simulink model "modelo_completo_codesys_final"  (R2020a)
settings: Solver=FixedStepAuto  StartTime=0.0  StopTime=inf  FixedStep=0.5e-3  MaxStep=1e-3  RelTol=1e-3
undefined symbols (not defined in the file): bac, baiz, bcx, bcy, Beqtran, Bheqd, bw, DiscIntNeverNeededParam, g, Kcy, ksac, ksaiz, ksiac, ksiaiz, Kw, lh0, Meq, Mheq, Rd, Rr, rt, rtd, xl0, xt0, yl0, yt0
libraries: simulink x13, powerlib_meascontrol x4, vrlib x2, dspswit3 x1
settings Model: SimulationMode=accelerator  Creator=tomas  LastModifiedBy=quiro
settings DataIOCC: ReturnWorkspaceOutputs=off
settings OptimizationCC: EfficientMapNaN2IntZero=off
settings DebuggingCC: ArithmeticOperatorsInVariantConditions=warning
settings HardwareCC: ProdBitPerPointer=32  ProdBitPerSizeT=32  ProdBitPerPtrDiffT=32  ProdWordSize=32  ProdHWDeviceType=Intel->x86-32 (Windows32)  TargetBitPerPointer=64  TargetBitPerSizeT=64  TargetBitPerPtrDiffT=64  TargetLongLongMode=on  TargetIntDivRoundTo=Zero  TargetEndianess=LittleEndian  TargetWordSize=64  TargetHWDeviceType=MATLAB Host  ProdEqTarget=off
settings SFSimCC: SimUseLocalCustomCode=off  CustomCodeUndefinedFunction=UseInterfaceOnly
settings RTWCC: RTWUseLocalCustomCode=off
settings CodeAppCC: MaxIdLength=128  StateflowObjectComments=on
settings GRTTargetCC: TargetLangStandard=C89/C90 (ANSI)  CombineOutputUpdateFcns=off  GRTInterface=on
settings SimscapeCC: SimscapeNormalizeSystem=off

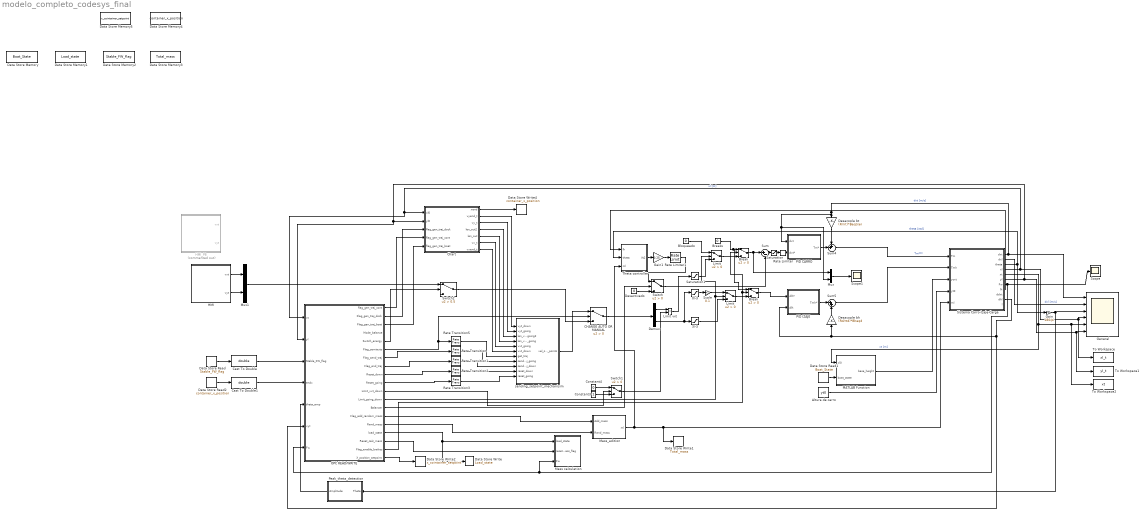
== system modelo_completo_codesys_final ==
  0/-3 : Saturate  UpperLimit=0.0  LowerLimit=-3.0
  3/-3 : Saturate  UpperLimit=3.0  LowerLimit=-3.0
  Altura de carro : Constant  Value=yt0
  Bloqueado : Constant  Value=0
  Break : Switch  Criteria=u2 > Threshold
  "Break " : Switch  Criteria=u2 > Threshold
  Breaks : Constant  Value=0
  CHANGE AUTO OR MANUAL : Switch  Criteria=u2 > Threshold
  Cast To Double : DataTypeConversion  OutDataTypeStr=double
  Cast To Double1 : DataTypeConversion  OutDataTypeStr=double
  Chart : Stateflow chart  TreatAsAtomicUnit=on
      settings: PortSchema="{\"entries\":[{\"content\":{\"sides\":[{\"content\":{\"connectorIds\":[\"In1\",\"In2\",\"In4\",\"In5\",\"In3\"]},\"type\":\"ConnectorPlacement.EquallySpacedRectSide\",\"uuid\":\"6b1ea9ed-88c8-4f45-af53-cf9c910626a6\"},{\"content\":{\"connectorIds\":[\"Out1\",\"Out2\",\"Out3\",\"Out4\",\"Out5\",\"Out6\",\"Out7\"],\"side\":\"RIGHT\"},\"type\":\"ConnectorPlacement.EquallySpacedRectSide\",\"uuid\":\"2b247f2b-a163-4c54-9e4e-ffcd144f96a2\"},{\"content\":{\"connectorIds\":[],\"side\":\"TOP\"},\"type\":\"ConnectorPlacement.EquallySpacedRectSide\",\"uuid\":\"aad476ba-6ce1-4a52-a412-e890bbacaba3\"}]},\"type\":\"ConnectorPlacement.EquallySpacedConnector\",\"uuid\":\"baf22a08-585d-4fcd-a6c0-f3cd3f47f06b\"}],\"packageUris\":[\"http://schema.mathworks.com/mf0/Connector/19700101\"],\"version\":\"1.0\"}"
  Constant3 : Constant
  Constant4 : Constant  Value=0
  Data Store Memory : DataStoreMemory  DataStoreName=Boat_State  ReadBeforeWriteMsg=warning  WriteAfterWriteMsg=warning  WriteAfterReadMsg=warning  InitialValue=[6;5;7;4;5; 4]  ShowAdditionalParam=off  OutDataTypeStr=double
  Data Store Memory1 : DataStoreMemory  DataStoreName=Load_state  ReadBeforeWriteMsg=warning  WriteAfterWriteMsg=warning  WriteAfterReadMsg=warning  ShowAdditionalParam=off  OutDataTypeStr=double
  Data Store Memory2 : DataStoreMemory  DataStoreName=Stable_FW_flag  ReadBeforeWriteMsg=warning  WriteAfterWriteMsg=warning  WriteAfterReadMsg=warning  ShowAdditionalParam=off  OutDataTypeStr=boolean
  Data Store Memory3 : DataStoreMemory  DataStoreName=Total_mass  ReadBeforeWriteMsg=warning  WriteAfterWriteMsg=warning  WriteAfterReadMsg=warning  InitialValue=15000.0  ShowAdditionalParam=off  OutDataTypeStr=double
  Data Store Memory4 : DataStoreMemory  DataStoreName=container_x_position  ReadBeforeWriteMsg=warning  WriteAfterWriteMsg=warning  WriteAfterReadMsg=warning  InitialValue=0.0  ShowAdditionalParam=off  OutDataTypeStr=double
  Data Store Memory5 : DataStoreMemory  DataStoreName=x_cointainer_setpoint  ReadBeforeWriteMsg=warning  WriteAfterWriteMsg=warning  WriteAfterReadMsg=warning  InitialValue=4  ShowAdditionalParam=off  OutDataTypeStr=double
  Data Store Read : DataStoreRead  DataStoreName=Stable_FW_flag
  Data Store Read1 : DataStoreRead  DataStoreName=Boat_State
  Data Store Read2 : DataStoreRead  DataStoreName=container_x_position  SampleTime=0.1
  Data Store Write : DataStoreWrite  DataStoreName=Load_state
  Data Store Write1 : DataStoreWrite  DataStoreName=Total_mass
  Data Store Write2 : DataStoreWrite  DataStoreName=x_cointainer_setpoint
  Data Store Write4 : DataStoreWrite  DataStoreName=container_x_position
  Demux : Demux  Outputs=2
  Desacople bh : Gain  Gain=(Rd/rtd)*Bheqd
  Desacople bt : Gain  Gain=(Rr/rt)*Beqtran
  Desactivado : Constant  Value=0
  Gain : Gain  Gain=180/pi
  Gain1 : Gain  Gain=0.25
  General : Scope  NumInputPorts=6
  HMI : Subsystem
  HMI_P8 : Subsystem  Commented=on
  Limit : Switch  Criteria=u2 > Threshold
  "Limit " : Switch  Criteria=u2 > Threshold
  Limit vxt : Product
  MATLAB Function : MATLAB Function  TreatAsAtomicUnit=on
  Mass calculation : Subsystem
  Mass_adition : Subsystem
  Mux : Mux  Inputs=2
  Mux1 : Mux  Inputs=2
  OPC READ/WRITE : Subsystem  TreatAsAtomicUnit=on  SystemSampleTime=0.1
  "PID CARRO " : Subsystem
  PID IZAJE : Subsystem
  Peak_theta_detection : Subsystem
  Rate Limiter : RateLimiter  SampleTimeMode=inherited
  Rate Limiter1 : RateLimiter  SampleTimeMode=inherited
  Rate Transition{,1..3,5} (5 alike) : RateTransition
  Saturation : Saturate  UpperLimit=4  LowerLimit=-4
  Saturation1 : Saturate  UpperLimit=4.0  LowerLimit=-4.0
  Scale : Gain  Gain=0.1
  Scope : Scope
  Scope1 : Scope
  "Sistema Carro-Izaje-Carga " : Subsystem
  Sum : Sum  Inputs=|+-
  Sum4 : Sum  Inputs=++|
  Sum5 : Sum  Inputs=|++
  Switch : Switch  Criteria=u2 > Threshold
  Switch1 : Switch  Criteria=u2 > Threshold
  Switch2 : Switch  Criteria=u2 > Threshold  Threshold=0.5
  Theta controller : Subsystem
  To Workspace : ToWorkspace  VariableName=xl_t  SampleTime=-1
  To Workspace1 : ToWorkspace  VariableName=yl_t  SampleTime=-1
  To Workspace2 : ToWorkspace  VariableName=xt  SampleTime=-1
  sending_setpoint_mechanisim : Subsystem
  wires:
  Sum4/1 -> "Sistema Carro-Izaje-Carga "/1(Tm)  "Tm***"
  Desacople bt/1 -> Sum4/1
  Desacople bh/1 -> Sum5/2
  PID IZAJE/1("Tmh* ") -> Sum5/1
  Switch/1 -> Sum/2
  Sum5/1 -> "Sistema Carro-Izaje-Carga "/2(Tmh)
  MATLAB Function/1(base_height) -> "Sistema Carro-Izaje-Carga "/3(ycxt)
  Altura de carro/1 -> "Sistema Carro-Izaje-Carga "/4(yt0)
  "Sistema Carro-Izaje-Carga "/1(dxt) -> General/1, "PID CARRO "/1(dxt), Mux/2, Desacople bt/1  "dxt [m/s]"
  "Sistema Carro-Izaje-Carga "/10(dhl) -> OPC READ/WRITE/6(vyt), PID IZAJE/2(dlh), Desacople bh/1
  Desactivado/1 -> Switch/3
  "Sistema Carro-Izaje-Carga "/8(lh) -> Theta controller/1(lh)
  "Sistema Carro-Izaje-Carga "/2(dxl) -> General/2  "dxl [m/s]"
  "Sistema Carro-Izaje-Carga "/3(theta) -> Theta controller/2(theta), Gain/1  "theta [rad]"
  "Sistema Carro-Izaje-Carga "/4(xl) -> OPC READ/WRITE/1(xt), Chart/1(xl0), General/4, To Workspace/1  "xl [m]"
  "Sistema Carro-Izaje-Carga "/5(xt) -> MATLAB Function/1(xl0), To Workspace2/1, General/5  "xt [m]"
  "PID CARRO "/1(Tm*) -> Sum4/2
  Gain/1 -> General/3, Peak_theta_detection/1(Theta)
  OPC READ/WRITE/13(Balancer) -> Switch/2
  HMI/1(vxt) -> Mux1/1
  HMI/2(vyt) -> Mux1/2
  OPC READ/WRITE/6(Flag_semiauto) -> CHANGE AUTO OR MANUAL/2, Rate Transition5/1
  CHANGE AUTO OR MANUAL/1 -> Demux/1
  Demux/2 -> 3/-3/1, 0/-3/1
  Peak_theta_detection/1(Amplitude) -> OPC READ/WRITE/5(theta_amp)
  OPC READ/WRITE/7(Flag_send_traj) -> Rate Transition/1
  OPC READ/WRITE/8(Flag_end_traj) -> Rate Transition1/1
  sending_setpoint_mechanisim/1(vel_sets_points) -> CHANGE AUTO OR MANUAL/1
  OPC READ/WRITE/10(Reset_going) -> Rate Transition3/1
  OPC READ/WRITE/9(Reset_down) -> Rate Transition2/1
  Saturation1/1 -> Limit/3
  "Limit "/1 -> "Break "/3
  0/-3/1 -> Scale/1
  Limit/1 -> Break/3
  Bloqueado/1 -> Limit/1
  Scale/1 -> "Limit "/1
  3/-3/1 -> "Limit "/3
  "Sistema Carro-Izaje-Carga "/7(Fw) -> Mass calculation/3(Fw), OPC READ/WRITE/7(Fw), Scope/1
  OPC READ/WRITE/11(Limit_vxt_down) -> Switch1/2
  Constant3/1 -> Switch1/3
  Constant4/1 -> Switch1/1
  Demux/1 -> Limit vxt/1
  Switch1/1 -> Limit vxt/2
  Limit vxt/1 -> Saturation1/1
  Data Store Read1/1 -> MATLAB Function/2(boat_state)
  Mass_adition/1(ml) -> Theta controller/3(ml), "Sistema Carro-Izaje-Carga "/5(ml), Data Store Write1/1
  OPC READ/WRITE/14(Flag_add_random_mass) -> Mass_adition/1(Add_mass)
  OPC READ/WRITE/15(Rand_mass) -> Mass_adition/2(Rand_mass)
  OPC READ/WRITE/17(Reset_calc_mass) -> Mass calculation/2(reset_mass_flag)
  Break/1 -> Mux/1, Sum/1
  "Break "/1 -> PID IZAJE/1(dlh*)
  Breaks/1 -> "Break "/1, Break/1
  OPC READ/WRITE/12(Limit_going_down) -> Limit/2, "Limit "/2
  Chart/6(vx_t) -> sending_setpoint_mechanisim/5(vxt_going)
  Chart/7(vxend_t) -> sending_setpoint_mechanisim/6(vxt_down)
  Chart/3(vy_t) -> sending_setpoint_mechanisim/2(vyt_going)
  Chart/2(vyend_t) -> sending_setpoint_mechanisim/1(vyt_down)
  Chart/4(len_out2) -> sending_setpoint_mechanisim/3(len_vec_going2)
  Chart/5(len_out) -> sending_setpoint_mechanisim/4(len_vec_going)
  OPC READ/WRITE/3(Flag_gen_traj_boat) -> Chart/3(flag_gen_traj_boat)
  OPC READ/WRITE/2(Flag_gen_traj_dock) -> Chart/4(flag_gen_traj_dock)
  "Sistema Carro-Izaje-Carga "/6(yl) -> General/6, To Workspace1/1, OPC READ/WRITE/2(yl), Chart/2(yl0)
  Data Store Read/1 -> Cast To Double/1
  Cast To Double/1 -> OPC READ/WRITE/3(Stable_FW_flag)
  Rate Transition/1 -> sending_setpoint_mechanisim/8(send_traj_going)
  Rate Transition1/1 -> sending_setpoint_mechanisim/9(send_traj_down)
  Rate Transition2/1 -> sending_setpoint_mechanisim/10(reset_down)
  Rate Transition3/1 -> sending_setpoint_mechanisim/11(reset_going)
  Rate Transition5/1 -> sending_setpoint_mechanisim/7(get_traj)
  Chart/1(xend) -> Data Store Write4/1
  Data Store Read2/1 -> Cast To Double1/1
  Cast To Double1/1 -> OPC READ/WRITE/4(endx)
  OPC READ/WRITE/18(Flag_enable_brakes) -> "Break "/2, Break/2
  OPC READ/WRITE/16(load_state) -> Data Store Write/1, Mass calculation/1(load_state)
  Switch2/1 -> CHANGE AUTO OR MANUAL/3
  Mux1/1 -> Switch2/1
  OPC READ/WRITE/5(Switch_energy) -> Switch2/2
  OPC READ/WRITE/19(X_position_setpoint) -> Data Store Write2/1
  OPC READ/WRITE/1(flag_gen_traj_cont) -> Chart/5(flag_gen_traj_cont)
  Gain1/1 -> Rate Limiter1/1
  Theta controller/1(Vt2) -> Gain1/1
  Rate Limiter1/1 -> Switch/1
  Sum/1 -> Saturation/1
  Saturation/1 -> Rate Limiter/1
  Rate Limiter/1 -> "PID CARRO "/2(dxt*)
  Mux/1 -> Scope1/1

== system modelo_completo_codesys_final/HMI ==
  Demux : Demux  Outputs=3
  First-Order Filter : powerlib_meascontrol/Filters/First-Order Filter  FilterType=Lowpass  Tc=10e-3  Ts=0  Initialize=off  Vac_Init=[0, 0, 60]  Vdc_Init=0  PlotResponse=off  FreqRange="[0,  200,  1]"
  First-Order Filter1 : powerlib_meascontrol/Filters/First-Order Filter  FilterType=Lowpass  Tc=10e-3  Ts=0  Initialize=off  Vac_Init=[0, 0, 60]  Vdc_Init=0  PlotResponse=off  FreqRange="[0,  200,  1]"
  Joystick Input : vrlib/Joystick Input  joyid=1  adjustports=on  forcefeed=off
  vxt : Outport
  vyt : Outport  Port=2
  wires:
  First-Order Filter1/1 -> vyt/1
  First-Order Filter/1 -> vxt/1
  Joystick Input/1 -> Demux/1
  Demux/1 -> First-Order Filter/1
  Demux/2 -> First-Order Filter1/1

== system modelo_completo_codesys_final/HMI_P8 ==
  Demux : Demux  Outputs=3
  Demux1 : Demux  Commented=on  Outputs=12
  First-Order Filter : powerlib_meascontrol/Filters/First-Order Filter  FilterType=Lowpass  Tc=10e-3  Ts=0  Initialize=off  Vac_Init=[0, 0, 60]  Vdc_Init=0  PlotResponse=off  FreqRange="[0,  200,  1]"
  First-Order Filter1 : powerlib_meascontrol/Filters/First-Order Filter  FilterType=Lowpass  Tc=10e-3  Ts=0  Initialize=off  Vac_Init=[0, 0, 60]  Vdc_Init=0  PlotResponse=off  FreqRange="[0,  200,  1]"
  Joystick Input : vrlib/Joystick Input  joyid=1  adjustports=on  forcefeed=off
  Scope : Scope  Commented=on  NumInputPorts=12
  Scope1 : Scope  NumInputPorts=2
  vxt : Outport
  vyt : Outport  Port=2
  wires:
  Joystick Input/1 -> Demux/1
  Demux1/12 -> Scope/12
  Demux1/11 -> Scope/11
  Demux1/10 -> Scope/10
  Demux1/9 -> Scope/9
  Demux1/8 -> Scope/8
  Demux1/7 -> Scope/7
  Demux1/6 -> Scope/6
  Demux1/5 -> Scope/5
  Demux1/4 -> Scope/4
  Demux1/3 -> Scope/3
  Demux1/2 -> Scope/2
  Demux1/1 -> Scope/1
  Demux/3 -> First-Order Filter1/1
  Demux/2 -> First-Order Filter/1
  Joystick Input/2 -> Demux1/1
  First-Order Filter/1 -> vxt/1, Scope1/1
  First-Order Filter1/1 -> vyt/1, Scope1/2

== system modelo_completo_codesys_final/Mass calculation ==
  load_state : Inport
  reset_mass_flag : Inport  Port=2
  Fw : Inport  Port=3
  Subsystem : Subsystem
  Subsystem1 : Subsystem
  wires:
  Fw/1 -> Subsystem1/1(Fw), Subsystem/1(Fw)
  load_state/1 -> Subsystem/Enable
  reset_mass_flag/1 -> Subsystem1/Enable, Subsystem/2(In1)

== system modelo_completo_codesys_final/Mass_adition ==
  Add_mass : Inport
  Rand_mass : Inport  Port=2
  Constant : Constant  Value=0
  Constant2 : Constant  Value=15000
  Sum1 : Sum
  add_random_mass : Switch  Criteria=u2 > Threshold
  ml : Outport
  wires:
  Add_mass/1 -> add_random_mass/2
  Constant/1 -> add_random_mass/3
  add_random_mass/1 -> Sum1/2
  Constant2/1 -> Sum1/1
  Sum1/1 -> ml/1
  Rand_mass/1 -> add_random_mass/1

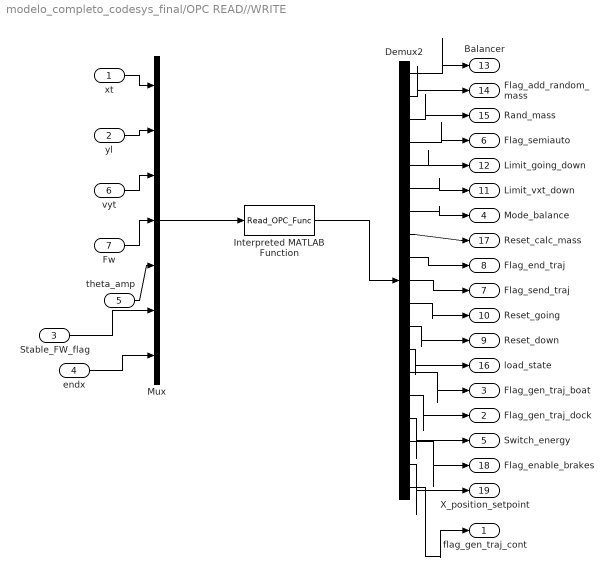
== system modelo_completo_codesys_final/OPC READ//WRITE ==
  xt : Inport
  yl : Inport  Port=2
  Stable_FW_flag : Inport  Port=3
  endx : Inport  Port=4
  theta_amp : Inport  Port=5
  vyt : Inport  Port=6
  Fw : Inport  Port=7
  Demux2 : Demux  Outputs=19
  Interpreted MATLAB Function : MATLABFcn  MATLABFcn=Read_OPC_Func
  Mux : Mux  Inputs=7
  flag_gen_traj_cont : Outport
  Flag_gen_traj_dock : Outport  Port=2
  Flag_gen_traj_boat : Outport  Port=3
  Mode_balance : Outport  Port=4
  Switch_energy : Outport  Port=5
  Flag_semiauto : Outport  Port=6
  Flag_send_traj : Outport  Port=7
  Flag_end_traj : Outport  Port=8
  Reset_down : Outport  Port=9
  Reset_going : Outport  Port=10
  Limit_vxt_down : Outport  Port=11
  Limit_going_down : Outport  Port=12
  Balancer : Outport  Port=13
  Flag_add_random_mass : Outport  Port=14
  Rand_mass : Outport  Port=15
  load_state : Outport  Port=16
  Reset_calc_mass : Outport  Port=17
  Flag_enable_brakes : Outport  Port=18
  X_position_setpoint : Outport  Port=19
  wires:
  Interpreted MATLAB Function/1 -> Demux2/1
  Stable_FW_flag/1 -> Mux/6
  Demux2/13 -> load_state/1
  Demux2/2 -> Flag_add_random_mass/1
  Demux2/12 -> Reset_down/1
  Demux2/11 -> Reset_going/1
  Demux2/9 -> Flag_end_traj/1
  Demux2/7 -> Mode_balance/1
  Demux2/3 -> Rand_mass/1
  Demux2/5 -> Limit_going_down/1
  Demux2/6 -> Limit_vxt_down/1
  Demux2/1 -> Balancer/1
  yl/1 -> Mux/2
  Mux/1 -> Interpreted MATLAB Function/1
  xt/1 -> Mux/1
  Demux2/8 -> Reset_calc_mass/1
  vyt/1 -> Mux/3
  Demux2/10 -> Flag_send_traj/1
  theta_amp/1 -> Mux/5
  Fw/1 -> Mux/4
  Demux2/4 -> Flag_semiauto/1
  Demux2/14 -> Flag_gen_traj_boat/1
  Demux2/15 -> Flag_gen_traj_dock/1
  endx/1 -> Mux/7
  Demux2/16 -> Switch_energy/1
  Demux2/17 -> Flag_enable_brakes/1
  Demux2/18 -> X_position_setpoint/1
  Demux2/19 -> flag_gen_traj_cont/1

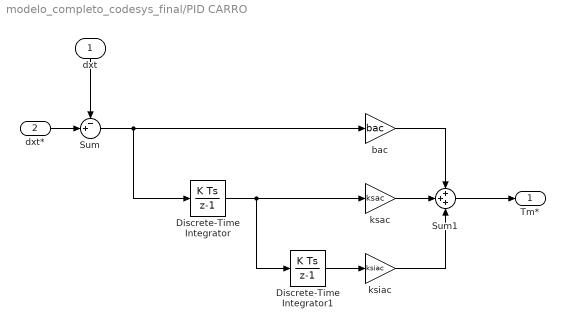
== system modelo_completo_codesys_final/PID CARRO  ==
  dxt : Inport
  dxt* : Inport  Port=2
  Discrete-Time Integrator : DiscreteIntegrator  SampleTime=-1  ICPrevOutput=DiscIntNeverNeededParam  ICPrevScaledInput=DiscIntNeverNeededParam
  Discrete-Time Integrator1 : DiscreteIntegrator  SampleTime=-1  ICPrevOutput=DiscIntNeverNeededParam  ICPrevScaledInput=DiscIntNeverNeededParam
  Sum : Sum  Inputs=-+|
  Sum1 : Sum  Inputs=+++
  bac : Gain  Gain=bac
  ksac : Gain  Gain=ksac
  ksiac : Gain  Gain=ksiac
  Tm* : Outport
  wires:
  dxt*/1 -> Sum/2
  dxt/1 -> Sum/1
  Sum1/1 -> Tm*/1
  bac/1 -> Sum1/1
  ksac/1 -> Sum1/2
  Discrete-Time Integrator1/1 -> ksiac/1
  ksiac/1 -> Sum1/3
  Sum/1 -> Discrete-Time Integrator/1, bac/1
  Discrete-Time Integrator/1 -> Discrete-Time Integrator1/1, ksac/1

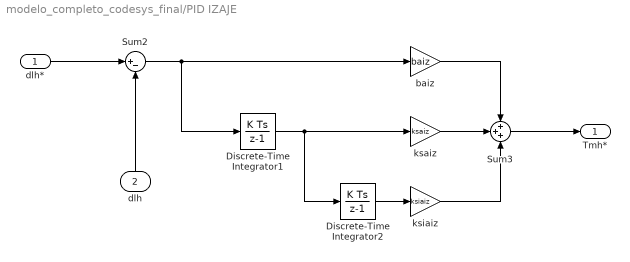
== system modelo_completo_codesys_final/PID IZAJE ==
  dlh* : Inport
  dlh : Inport  Port=2
  Discrete-Time Integrator1 : DiscreteIntegrator  SampleTime=-1  ICPrevOutput=DiscIntNeverNeededParam  ICPrevScaledInput=DiscIntNeverNeededParam
  Discrete-Time Integrator2 : DiscreteIntegrator  SampleTime=-1  ICPrevOutput=DiscIntNeverNeededParam  ICPrevScaledInput=DiscIntNeverNeededParam
  Sum2 : Sum  Inputs=|+-
  Sum3 : Sum  Inputs=+++
  baiz : Gain  Gain=baiz
  ksaiz : Gain  Gain=ksaiz
  ksiaiz : Gain  Gain=ksiaiz
  "Tmh* " : Outport
  wires:
  dlh/1 -> Sum2/2
  Sum3/1 -> "Tmh* "/1
  ksaiz/1 -> Sum3/2
  Discrete-Time Integrator2/1 -> ksiaiz/1
  baiz/1 -> Sum3/1
  ksiaiz/1 -> Sum3/3
  dlh*/1 -> Sum2/1
  Sum2/1 -> Discrete-Time Integrator1/1, baiz/1
  Discrete-Time Integrator1/1 -> Discrete-Time Integrator2/1, ksaiz/1

== system modelo_completo_codesys_final/Peak_theta_detection ==
  Theta : Inport
  Detect Decrease : simulink/Logic and Bit Operations/Detect Decrease  vinit=0.0  OutDataTypeStr=boolean
  Detect Rise Positive : simulink/Logic and Bit Operations/Detect Rise Positive  vinit=0  OutDataTypeStr=boolean
  MinMax Running Resettable : simulink/Math Operations/MinMax Running Resettable  Function=max  vinit=0.0
  Subsystem : Subsystem
  Amplitude : Outport
  wires:
  Theta/1 -> Detect Decrease/1, Detect Rise Positive/1, MinMax Running Resettable/1
  Subsystem/1(Out1) -> Amplitude/1
  MinMax Running Resettable/1 -> Subsystem/1(In1)
  Detect Rise Positive/1 -> MinMax Running Resettable/2
  Detect Decrease/1 -> Subsystem/Trigger

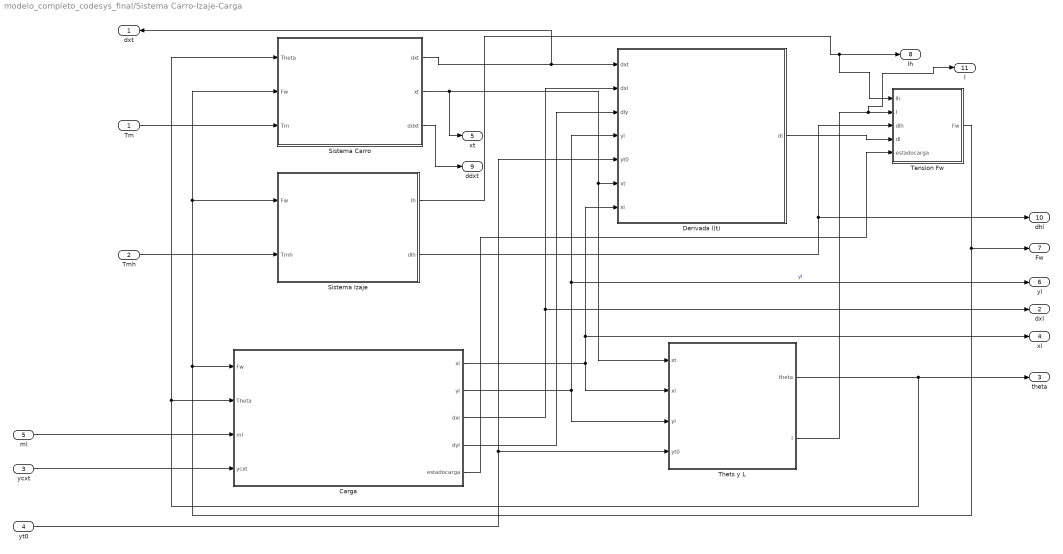
== system modelo_completo_codesys_final/Sistema Carro-Izaje-Carga  ==
  Tm : Inport
  Tmh : Inport  Port=2
  ycxt : Inport  Port=3
  yt0 : Inport  Port=4
  ml : Inport  Port=5
  "Carga " : Subsystem
  Derivada l(t) : Subsystem
  Sistema Carro : Subsystem
  Sistema Izaje : Subsystem
  Tension Fw : Subsystem
  Thets y L : Subsystem
  dxt : Outport
  dxl : Outport  Port=2
  theta : Outport  Port=3
  xl : Outport  Port=4
  xt : Outport  Port=5
  yl : Outport  Port=6
  Fw : Outport  Port=7
  lh : Outport  Port=8
  ddxt : Outport  Port=9
  dhl : Outport  Port=10
  l : Outport  Port=11
  wires:
  Sistema Izaje/1(lh) -> Tension Fw/1(lh), lh/1
  Sistema Izaje/2(dlh) -> dhl/1, Tension Fw/3(dlh)
  "Carga "/2(yl) -> yl/1, Derivada l(t)/4(yl), Thets y L/3(yl)  "yl"
  "Carga "/3(dxl) -> dxl/1, Derivada l(t)/2(dxl)
  "Carga "/4(dyl) -> Derivada l(t)/3(dly)
  Derivada l(t)/1(dl) -> Tension Fw/4(dl)
  Thets y L/1("theta ") -> theta/1, Sistema Carro/1(Theta), "Carga "/2(Theta)
  ml/1 -> "Carga "/3(ml)
  ycxt/1 -> "Carga "/4(ycxt)
  "Carga "/5("estadocarga ") -> Tension Fw/5(estadocarga)
  Thets y L/2("l ") -> l/1, Tension Fw/2(l)
  Tm/1 -> Sistema Carro/3(Tm)
  Tmh/1 -> Sistema Izaje/2(Tmh)
  yt0/1 -> Derivada l(t)/5(yt0), Thets y L/4(yt0)
  "Carga "/1(xl) -> Derivada l(t)/7(xl), xl/1, Thets y L/2(xl)
  Tension Fw/1("Fw ") -> Fw/1, Sistema Carro/2(Fw), Sistema Izaje/1(Fw), "Carga "/1(Fw)
  Sistema Carro/3("ddxt ") -> ddxt/1
  Sistema Carro/2(xt) -> xt/1, Derivada l(t)/6(xt), Thets y L/1(xt)
  Sistema Carro/1("dxt ") -> Derivada l(t)/1(dxt), dxt/1

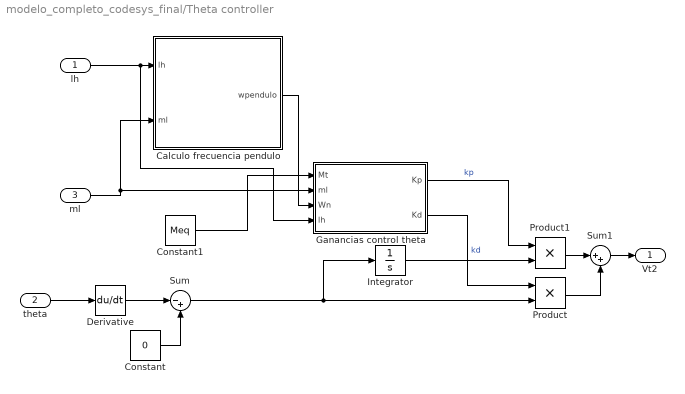
== system modelo_completo_codesys_final/Theta controller ==
  lh : Inport
  theta : Inport  Port=2
  ml : Inport  Port=3
  Calculo frecuencia pendulo : Subsystem
  Constant : Constant  Value=0
  Constant1 : Constant  Value=Meq
  Derivative : Derivative
  Ganancias control theta : MATLAB Function  TreatAsAtomicUnit=on
  Integrator : Integrator
  Product : Product
  Product1 : Product
  Sum : Sum  Inputs=|-+
  Sum1 : Sum  Inputs=|++
  Vt2 : Outport
  wires:
  Product1/1 -> Sum1/1
  theta/1 -> Derivative/1
  Product/1 -> Sum1/2
  Sum/1 -> Integrator/1, Product/2
  Ganancias control theta/1(Kp) -> Product1/1  "kp"
  Ganancias control theta/2(Kd) -> Product/1  "kd"
  Constant/1 -> Sum/2
  lh/1 -> Ganancias control theta/4(lh), Calculo frecuencia pendulo/1(lh)
  ml/1 -> Calculo frecuencia pendulo/2(ml), Ganancias control theta/2(ml)
  Sum1/1 -> Vt2/1
  Calculo frecuencia pendulo/1("wpendulo ") -> Ganancias control theta/3(Wn)
  Constant1/1 -> Ganancias control theta/1(Mt)
  Derivative/1 -> Sum/1
  Integrator/1 -> Product1/2

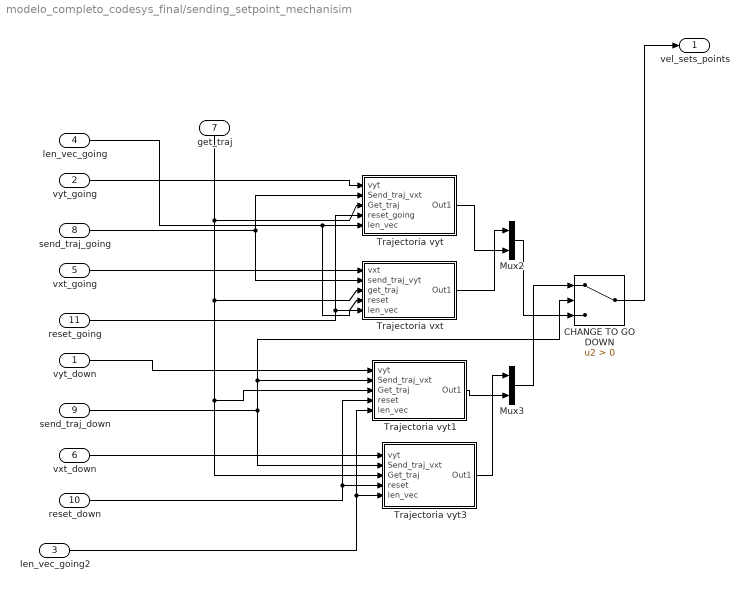
== system modelo_completo_codesys_final/sending_setpoint_mechanisim ==
  vyt_down : Inport
  vyt_going : Inport  Port=2
  len_vec_going2 : Inport  Port=3
  len_vec_going : Inport  Port=4
  vxt_going : Inport  Port=5
  vxt_down : Inport  Port=6
  get_traj : Inport  Port=7
  send_traj_going : Inport  Port=8
  send_traj_down : Inport  Port=9
  reset_down : Inport  Port=10
  reset_going : Inport  Port=11
  CHANGE TO GO DOWN : Switch  Criteria=u2 > Threshold
  Mux2 : Mux  Inputs=2
  Mux3 : Mux  Inputs=2
  Trajectoria vxt : Subsystem
  Trajectoria vyt : Subsystem
  Trajectoria vyt1 : Subsystem
  Trajectoria vyt3 : Subsystem
  vel_sets_points : Outport
  wires:
  get_traj/1 -> Trajectoria vyt3/3(Get_traj), Trajectoria vyt1/3(Get_traj), Trajectoria vxt/3("get_traj "), Trajectoria vyt/3(Get_traj)
  vyt_going/1 -> Trajectoria vyt/1("vyt ")
  Trajectoria vxt/1(Out1) -> Mux2/1
  Trajectoria vyt/1(Out1) -> Mux2/2
  vxt_going/1 -> Trajectoria vxt/1(vxt)
  send_traj_going/1 -> Trajectoria vxt/2(send_traj_vyt), Trajectoria vyt/2("Send_traj_vxt ")
  vyt_down/1 -> Trajectoria vyt1/1("vyt ")
  vxt_down/1 -> Trajectoria vyt3/1("vyt ")
  send_traj_down/1 -> Trajectoria vyt3/2("Send_traj_vxt "), Trajectoria vyt1/2("Send_traj_vxt "), CHANGE TO GO DOWN/2
  Trajectoria vyt1/1(Out1) -> Mux3/2
  Trajectoria vyt3/1(Out1) -> Mux3/1
  CHANGE TO GO DOWN/1 -> vel_sets_points/1
  Mux3/1 -> CHANGE TO GO DOWN/1
  Mux2/1 -> CHANGE TO GO DOWN/3
  reset_going/1 -> Trajectoria vxt/4(reset), Trajectoria vyt/4(reset_going)
  reset_down/1 -> Trajectoria vyt3/4(reset), Trajectoria vyt1/4(reset)
  len_vec_going/1 -> Trajectoria vxt/5(len_vec), Trajectoria vyt/5(len_vec)
  len_vec_going2/1 -> Trajectoria vyt3/5(len_vec), Trajectoria vyt1/5(len_vec)

== system modelo_completo_codesys_final/Mass calculation/Subsystem ==
  Fw : Inport
  In1 : Inport  Port=2
  Enable : EnablePort  StatesWhenEnabling=reset
  Data Store Write : DataStoreWrite  DataStoreName=Stable_FW_flag
  Data Store Write1 : DataStoreWrite  Commented=on  DataStoreName=Total_mass
  Gain : Gain  Gain=1/9.81
  Subsystem : Subsystem
  wires:
  Fw/1 -> Subsystem/1(Fw)
  Subsystem/1(Mass) -> Gain/1
  Subsystem/2(Stable_Fw_flag) -> Data Store Write/1
  In1/1 -> Subsystem/Reset
  Gain/1 -> Data Store Write1/1

== system modelo_completo_codesys_final/Mass calculation/Subsystem1 ==
  Fw : Inport
  Enable : EnablePort
  Data Store Write : DataStoreWrite  DataStoreName=Stable_FW_flag
  Peak_theta_detection1 : Subsystem  TreatAsAtomicUnit=on  SystemSampleTime=0.1
  wires:
  Fw/1 -> Peak_theta_detection1/1(Fw)
  Peak_theta_detection1/1(Logical_output) -> Data Store Write/1

== system modelo_completo_codesys_final/Peak_theta_detection/Subsystem ==
  In1 : Inport
  Trigger : TriggerPort  VariantControl=Variant  PortDimensions=1
  Out1 : Outport
  wires:
  In1/1 -> Out1/1

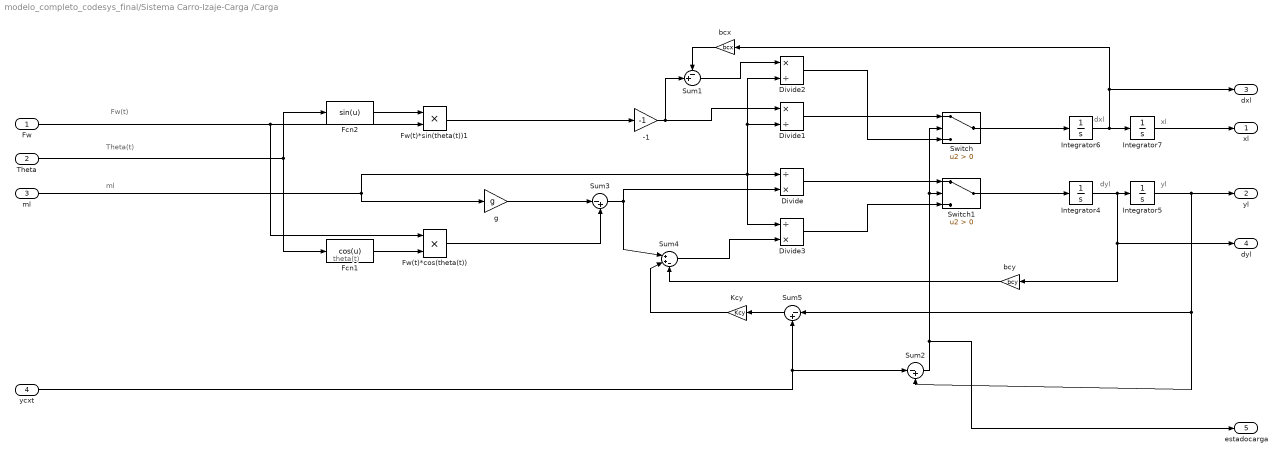
== system modelo_completo_codesys_final/Sistema Carro-Izaje-Carga /Carga  ==
  note: Theta(t)
  note: Fw(t)
  note: ml
  note: theta(t)
  note: dyl
  note: yl
  note: dxl
  note: xl
  Fw : Inport
  Theta : Inport  Port=2
  ml : Inport  Port=3
  ycxt : Inport  Port=4
  -1 : Gain  Gain=-1
  Divide : Product  Inputs=/*
  Divide1 : Product  Inputs=*/
  Divide2 : Product  Inputs=*/
  Divide3 : Product  Inputs=/*
  Fcn1 : Fcn  Expr=cos(u)
  Fcn2 : Fcn  Expr=sin(u)
  Fw(t)*cos(theta(t)) : Product
  Fw(t)*sin(theta(t))1 : Product
  Integrator4 : Integrator
  Integrator5 : Integrator  InitialCondition=yl0
  Integrator6 : Integrator
  Integrator7 : Integrator  InitialCondition=xl0
  Kcy : Gain  Gain=Kcy
  Sum1 : Sum  Inputs=-+|
  Sum2 : Sum  Inputs=|-+
  Sum3 : Sum  Inputs=|-+
  Sum4 : Sum  Inputs=|++-
  Sum5 : Sum  Inputs=|-+
  Switch : Switch  Criteria=u2 > Threshold
  Switch1 : Switch  Criteria=u2 > Threshold
  bcx : Gain  Gain=bcx
  bcy : Gain  Gain=bcy
  g : Gain  Gain=g
  xl : Outport
  yl : Outport  Port=2
  dxl : Outport  Port=3
  dyl : Outport  Port=4
  "estadocarga " : Outport  Port=5
  wires:
  Fcn2/1 -> Fw(t)*sin(theta(t))1/1
  Theta/1 -> Fcn1/1, Fcn2/1
  g/1 -> Sum3/1
  Fcn1/1 -> Fw(t)*cos(theta(t))/2
  Fw(t)*cos(theta(t))/1 -> Sum3/2
  Fw/1 -> Fw(t)*cos(theta(t))/1, Fw(t)*sin(theta(t))1/2
  ml/1 -> Divide1/2, Divide2/2, Divide3/1, Divide/1, g/1
  Integrator7/1 -> xl/1
  Integrator6/1 -> Integrator7/1, dxl/1, bcx/1
  Fw(t)*sin(theta(t))1/1 -> -1/1
  Integrator5/1 -> Sum2/2, Sum5/1, yl/1
  Divide1/1 -> Switch/1
  -1/1 -> Sum1/2, Divide1/1
  Integrator4/1 -> dyl/1, bcy/1, Integrator5/1
  Sum3/1 -> Sum4/1, Divide/2
  Switch/1 -> Integrator6/1
  bcx/1 -> Sum1/1
  Sum2/1 -> "estadocarga "/1, Switch1/2, Switch/2
  ycxt/1 -> Sum2/1, Sum5/2
  Sum1/1 -> Divide2/1
  Divide2/1 -> Switch/3
  Sum4/1 -> Divide3/2
  Divide3/1 -> Switch1/3
  Switch1/1 -> Integrator4/1
  Divide/1 -> Switch1/1
  Sum5/1 -> Kcy/1
  Kcy/1 -> Sum4/2
  bcy/1 -> Sum4/3

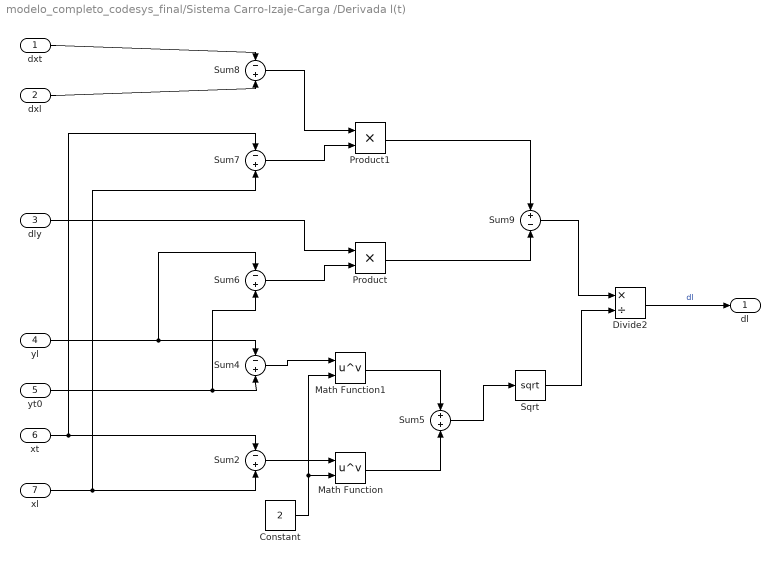
== system modelo_completo_codesys_final/Sistema Carro-Izaje-Carga /Derivada l(t) ==
  dxt : Inport
  dxl : Inport  Port=2
  dly : Inport  Port=3
  yl : Inport  Port=4
  yt0 : Inport  Port=5
  xt : Inport  Port=6
  xl : Inport  Port=7
  Constant : Constant  Value=2
  Divide2 : Product  Inputs=*/
  Math Function : Math  Operator=pow  SignedPower=on  SaturateOnIntegerOverflow=on
  Math Function1 : Math  Operator=pow  SignedPower=on  SaturateOnIntegerOverflow=on
  Product : Product
  Product1 : Product
  Sqrt : Sqrt  SaturateOnIntegerOverflow=on
  Sum{2,4,6..8} (5 alike) : Sum  Inputs=-+
  Sum5 : Sum
  Sum9 : Sum  Inputs=+-
  dl : Outport
  wires:
  Divide2/1 -> dl/1  "dl"
  dly/1 -> Product/1
  yl/1 -> Sum6/1, Sum4/1
  xl/1 -> Sum7/2, Sum2/2
  Product/1 -> Sum9/2
  dxt/1 -> Sum8/1
  Sum5/1 -> Sqrt/1
  Constant/1 -> Math Function1/2, Math Function/2
  yt0/1 -> Sum4/2, Sum6/2
  dxl/1 -> Sum8/2
  Math Function1/1 -> Sum5/1
  Sum8/1 -> Product1/1
  Sum9/1 -> Divide2/1
  Math Function/1 -> Sum5/2
  xt/1 -> Sum7/1, Sum2/1
  Sum6/1 -> Product/2
  Sum7/1 -> Product1/2
  Product1/1 -> Sum9/1
  Sum4/1 -> Math Function1/1
  Sqrt/1 -> Divide2/2
  Sum2/1 -> Math Function/1

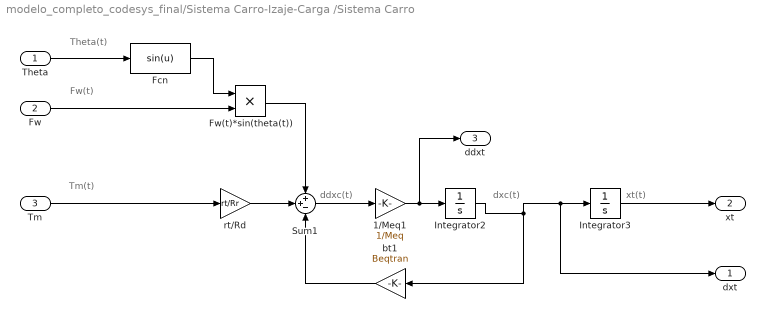
== system modelo_completo_codesys_final/Sistema Carro-Izaje-Carga /Sistema Carro ==
  note: dxc(t)
  note: xt(t)
  note: ddxc(t)
  note: Theta(t)
  note: Fw(t)
  note: Tm(t)
  Theta : Inport
  Fw : Inport  Port=2
  Tm : Inport  Port=3
  1/Meq1 : Gain  Gain=1/Meq
  Fcn : Fcn  Expr=sin(u)
  Fw(t)*sin(theta(t)) : Product
  Integrator2 : Integrator
  Integrator3 : Integrator  InitialCondition=xt0
  Sum1 : Sum  Inputs=++-
  bt1 : Gain  Gain=Beqtran
  rt/Rd : Gain  Gain=rt/Rr
  "dxt " : Outport
  xt : Outport  Port=2
  "ddxt " : Outport  Port=3
  wires:
  Integrator3/1 -> xt/1
  Sum1/1 -> 1/Meq1/1
  Fw/1 -> Fw(t)*sin(theta(t))/2
  Fcn/1 -> Fw(t)*sin(theta(t))/1
  rt/Rd/1 -> Sum1/2
  Theta/1 -> Fcn/1
  Fw(t)*sin(theta(t))/1 -> Sum1/1
  1/Meq1/1 -> "ddxt "/1, Integrator2/1
  Tm/1 -> rt/Rd/1
  bt1/1 -> Sum1/3
  Integrator2/1 -> "dxt "/1, Integrator3/1, bt1/1

== system modelo_completo_codesys_final/Sistema Carro-Izaje-Carga /Sistema Izaje ==
  note: lh(t)
  note: dlh(t)
  note: ddlh(t)
  note: Tmh(t)
  note: Fw(t)
  Fw : Inport
  Tmh : Inport  Port=2
  1/Meq : Gain  Gain=1/Mheq
  Integrator : Integrator
  Integrator1 : Integrator  InitialCondition=lh0
  Sum : Sum  Inputs=++-
  bt : Gain  Gain=Bheqd
  rtd/Rd : Gain  Gain=-rtd/Rd
  lh : Outport
  dlh : Outport  Port=2
  wires:
  Integrator/1 -> dlh/1, bt/1, Integrator1/1
  Integrator1/1 -> lh/1
  rtd/Rd/1 -> Sum/2
  bt/1 -> Sum/3
  Fw/1 -> Sum/1
  Tmh/1 -> rtd/Rd/1
  1/Meq/1 -> Integrator/1
  Sum/1 -> 1/Meq/1

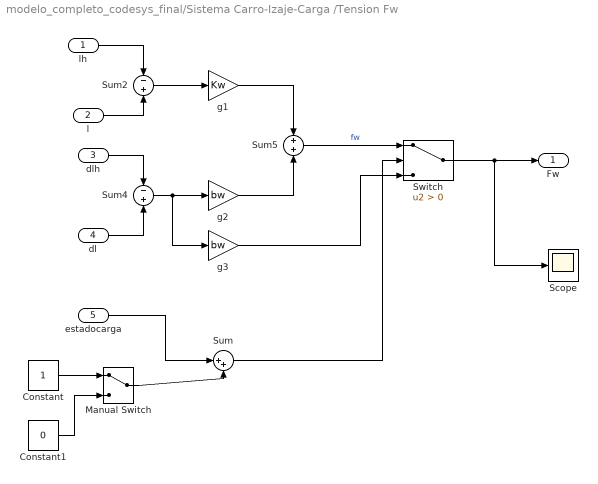
== system modelo_completo_codesys_final/Sistema Carro-Izaje-Carga /Tension Fw ==
  lh : Inport
  l : Inport  Port=2
  dlh : Inport  Port=3
  dl : Inport  Port=4
  estadocarga : Inport  Port=5
  Constant : Constant
  Constant1 : Constant  Value=0
  Manual Switch : ManualSwitch
  Scope : Scope
  Sum : Sum  Inputs=|++
  Sum2 : Sum  Inputs=-+
  Sum4 : Sum  Inputs=-+
  Sum5 : Sum
  Switch : Switch  Criteria=u2 > Threshold
  g1 : Gain  Gain=Kw
  g2 : Gain  Gain=bw
  g3 : Gain  Gain=bw
  "Fw " : Outport
  wires:
  l/1 -> Sum2/2
  dl/1 -> Sum4/2
  g2/1 -> Sum5/2
  Sum5/1 -> Switch/1  "fw"
  Sum4/1 -> g3/1, g2/1
  g1/1 -> Sum5/1
  dlh/1 -> Sum4/1
  g3/1 -> Switch/3
  lh/1 -> Sum2/1
  Switch/1 -> Scope/1, "Fw "/1
  Sum2/1 -> g1/1
  Constant/1 -> Manual Switch/1
  Constant1/1 -> Manual Switch/2
  Manual Switch/1 -> Sum/2
  estadocarga/1 -> Sum/1
  Sum/1 -> Switch/2

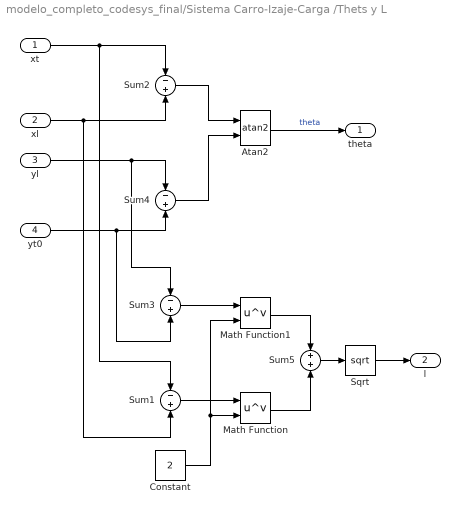
== system modelo_completo_codesys_final/Sistema Carro-Izaje-Carga /Thets y L ==
  xt : Inport
  xl : Inport  Port=2
  yl : Inport  Port=3
  yt0 : Inport  Port=4
  Atan2 : Trigonometry  Operator=atan2
  Constant : Constant  Value=2
  Math Function : Math  Operator=pow  SignedPower=on  SaturateOnIntegerOverflow=on
  Math Function1 : Math  Operator=pow  SignedPower=on  SaturateOnIntegerOverflow=on
  Sqrt : Sqrt  SaturateOnIntegerOverflow=on
  Sum{1..4} (4 alike) : Sum  Inputs=-+
  Sum5 : Sum
  "theta " : Outport
  "l " : Outport  Port=2
  wires:
  Sum4/1 -> Atan2/2
  xt/1 -> Sum1/1, Sum2/1
  xl/1 -> Sum1/2, Sum2/2
  yt0/1 -> Sum3/2, Sum4/2
  Atan2/1 -> "theta "/1  "theta"
  yl/1 -> Sum3/1, Sum4/1
  Sum2/1 -> Atan2/1
  Sqrt/1 -> "l "/1
  Math Function/1 -> Sum5/2
  Math Function1/1 -> Sum5/1
  Sum3/1 -> Math Function1/1
  Sum1/1 -> Math Function/1
  Constant/1 -> Math Function/2, Math Function1/2
  Sum5/1 -> Sqrt/1

== system modelo_completo_codesys_final/Theta controller/Calculo frecuencia pendulo ==
  lh : Inport
  ml : Inport  Port=2
  Constant : Constant  Value=Meq*9.81
  Constant1 : Constant  Value=Meq
  Divide : Product  Inputs=*/
  Product : Product
  Sqrt : Sqrt  OutputSignalType=real  SaturateOnIntegerOverflow=on
  Sum : Sum  Inputs=++|
  "wpendulo " : Outport
  wires:
  Divide/1 -> Sqrt/1
  Sqrt/1 -> "wpendulo "/1
  Constant/1 -> Divide/1
  Sum/1 -> Product/1
  Constant1/1 -> Sum/1
  ml/1 -> Sum/2
  lh/1 -> Product/2
  Product/1 -> Divide/2

== system modelo_completo_codesys_final/sending_setpoint_mechanisim/Trajectoria vxt ==
  vxt : Inport
  send_traj_vyt : Inport  Port=2
  "get_traj " : Inport  Port=3
  reset : Inport  Port=4
  len_vec : Inport  Port=5
  Subsystem2 : Subsystem
  Subsystem3 : Subsystem
  Out1 : Outport
  wires:
  vxt/1 -> Subsystem2/1(In1)
  Subsystem2/1(Out1) -> Subsystem3/1(In1)
  send_traj_vyt/1 -> Subsystem3/Enable
  Subsystem3/1(Out1) -> Out1/1
  "get_traj "/1 -> Subsystem2/Enable
  reset/1 -> Subsystem3/2(In2)
  len_vec/1 -> Subsystem3/3(In3)

== system modelo_completo_codesys_final/sending_setpoint_mechanisim/Trajectoria vyt ==
  "vyt " : Inport
  "Send_traj_vxt " : Inport  Port=2
  Get_traj : Inport  Port=3
  reset_going : Inport  Port=4
  len_vec : Inport  Port=5
  Subsystem2 : Subsystem
  Subsystem3 : Subsystem
  Out1 : Outport
  wires:
  "vyt "/1 -> Subsystem2/1(In1)
  Subsystem2/1(Out1) -> Subsystem3/1(In1)
  "Send_traj_vxt "/1 -> Subsystem3/Enable
  Subsystem3/1(Out1) -> Out1/1
  Get_traj/1 -> Subsystem2/Enable
  reset_going/1 -> Subsystem3/2(In2)
  len_vec/1 -> Subsystem3/3(In3)

== system modelo_completo_codesys_final/sending_setpoint_mechanisim/Trajectoria vyt1 ==
  "vyt " : Inport
  "Send_traj_vxt " : Inport  Port=2
  Get_traj : Inport  Port=3
  reset : Inport  Port=4
  len_vec : Inport  Port=5
  Subsystem2 : Subsystem
  Subsystem3 : Subsystem
  Out1 : Outport
  wires:
  "vyt "/1 -> Subsystem2/1(In1)
  Subsystem2/1(Out1) -> Subsystem3/1(In1)
  "Send_traj_vxt "/1 -> Subsystem3/Enable
  Subsystem3/1(Out1) -> Out1/1
  Get_traj/1 -> Subsystem2/Enable
  reset/1 -> Subsystem3/2(In2)
  len_vec/1 -> Subsystem3/3(In3)

== system modelo_completo_codesys_final/sending_setpoint_mechanisim/Trajectoria vyt3 ==
  "vyt " : Inport
  "Send_traj_vxt " : Inport  Port=2
  Get_traj : Inport  Port=3
  reset : Inport  Port=4
  len_vec : Inport  Port=5
  Subsystem2 : Subsystem
  Subsystem3 : Subsystem
  Out1 : Outport
  wires:
  "vyt "/1 -> Subsystem2/1(In1)
  Subsystem2/1(Out1) -> Subsystem3/1(In1)
  "Send_traj_vxt "/1 -> Subsystem3/Enable
  Subsystem3/1(Out1) -> Out1/1
  Get_traj/1 -> Subsystem2/Enable
  reset/1 -> Subsystem3/2(In2)
  len_vec/1 -> Subsystem3/3(In3)

== system modelo_completo_codesys_final/Mass calculation/Subsystem/Subsystem ==
  Fw : Inport
  Reset : ResetPort  DisableCoverage=on  ResetTriggerType=either
  Gain : Gain  Gain=1/9.81
  Peak_theta_detection1 : Subsystem  TreatAsAtomicUnit=on  SystemSampleTime=0.1
  Mass : Outport
  Stable_Fw_flag : Outport  Port=2
  wires:
  Gain/1 -> Mass/1
  Fw/1 -> Peak_theta_detection1/1(Fw)
  Peak_theta_detection1/1(Amplitude) -> Gain/1
  Peak_theta_detection1/2(Logical_output) -> Stable_Fw_flag/1

== system modelo_completo_codesys_final/Mass calculation/Subsystem1/Peak_theta_detection1 ==
  Fw : Inport
  Compare To Constant : simulink/Logic and Bit Operations/Compare To Constant  relop=>=  const=14000*9.8  OutDataTypeStr=boolean
  Detect Decrease : simulink/Logic and Bit Operations/Detect Decrease  vinit=0.0  OutDataTypeStr=boolean
  Detect Increase : simulink/Logic and Bit Operations/Detect Increase  vinit=0.0  OutDataTypeStr=boolean
  Detect Rise Positive : simulink/Logic and Bit Operations/Detect Rise Positive  vinit=0  OutDataTypeStr=boolean
  Logical Operator : Logic  AllPortsSameDT=off  OutDataTypeStr=boolean
  MinMax Running Resettable : simulink/Math Operations/MinMax Running Resettable  Function=max  vinit=0.0
  Scope : Scope
  Subsystem : Subsystem
  Logical_output : Outport
  wires:
  Fw/1 -> Detect Decrease/1, Detect Rise Positive/1, MinMax Running Resettable/1
  MinMax Running Resettable/1 -> Subsystem/1(In1)
  Detect Rise Positive/1 -> MinMax Running Resettable/2
  Detect Decrease/1 -> Subsystem/Trigger
  Detect Increase/1 -> Logical Operator/1
  Subsystem/1(Out1) -> Scope/1, Compare To Constant/1, Detect Increase/1
  Logical Operator/1 -> Logical_output/1
  Compare To Constant/1 -> Logical Operator/2

== system modelo_completo_codesys_final/sending_setpoint_mechanisim/Trajectoria vxt/Subsystem2 ==
  In1 : Inport
  Enable : EnablePort
  Out1 : Outport
  wires:
  In1/1 -> Out1/1

== system modelo_completo_codesys_final/sending_setpoint_mechanisim/Trajectoria vxt/Subsystem3 ==
  In1 : Inport
  In2 : Inport  Port=2
  In3 : Inport  Port=3
  Enable : EnablePort
  Resettable Subsystem : Subsystem  TreatAsAtomicUnit=on
  Out1 : Outport
  wires:
  In1/1 -> Resettable Subsystem/1(In1)
  In2/1 -> Resettable Subsystem/Reset
  Resettable Subsystem/1(Out1) -> Out1/1
  In3/1 -> Resettable Subsystem/2(len_vector)

== system modelo_completo_codesys_final/sending_setpoint_mechanisim/Trajectoria vyt/Subsystem2 ==
  In1 : Inport
  Enable : EnablePort
  Out1 : Outport
  wires:
  In1/1 -> Out1/1

== system modelo_completo_codesys_final/sending_setpoint_mechanisim/Trajectoria vyt/Subsystem3 ==
  In1 : Inport
  In2 : Inport  Port=2
  In3 : Inport  Port=3
  Enable : EnablePort
  Resettable Subsystem : Subsystem  TreatAsAtomicUnit=on
  Out1 : Outport
  wires:
  In1/1 -> Resettable Subsystem/1(In1)
  In2/1 -> Resettable Subsystem/Reset
  Resettable Subsystem/1(Out1) -> Out1/1
  In3/1 -> Resettable Subsystem/2(len_vector)

== system modelo_completo_codesys_final/sending_setpoint_mechanisim/Trajectoria vyt1/Subsystem2 ==
  In1 : Inport
  Enable : EnablePort
  Out1 : Outport
  wires:
  In1/1 -> Out1/1

== system modelo_completo_codesys_final/sending_setpoint_mechanisim/Trajectoria vyt1/Subsystem3 ==
  In1 : Inport
  In2 : Inport  Port=2
  In3 : Inport  Port=3
  Enable : EnablePort
  Resettable Subsystem : Subsystem  TreatAsAtomicUnit=on
  Out1 : Outport
  wires:
  In1/1 -> Resettable Subsystem/1(In1)
  In2/1 -> Resettable Subsystem/Reset
  Resettable Subsystem/1(Out1) -> Out1/1
  In3/1 -> Resettable Subsystem/2(len_vector)

== system modelo_completo_codesys_final/sending_setpoint_mechanisim/Trajectoria vyt3/Subsystem2 ==
  In1 : Inport
  Enable : EnablePort
  Out1 : Outport
  wires:
  In1/1 -> Out1/1

== system modelo_completo_codesys_final/sending_setpoint_mechanisim/Trajectoria vyt3/Subsystem3 ==
  In1 : Inport
  In2 : Inport  Port=2
  In3 : Inport  Port=3
  Enable : EnablePort
  Resettable Subsystem : Subsystem  TreatAsAtomicUnit=on
  Out1 : Outport
  wires:
  In1/1 -> Resettable Subsystem/1(In1)
  In2/1 -> Resettable Subsystem/Reset
  Resettable Subsystem/1(Out1) -> Out1/1
  In3/1 -> Resettable Subsystem/2(len_vector)

== system modelo_completo_codesys_final/Mass calculation/Subsystem/Subsystem/Peak_theta_detection1 ==
  Fw : Inport
  Compare To Constant1 : simulink/Logic and Bit Operations/Compare To Constant  relop=>=  const=2  OutDataTypeStr=boolean
  Counter : dspswit3/Counter  Direction=Up  CountEvent=Rising edge  CounterSize=8 bits  MaxCount=2  InitialCount=0  Output=Count  HitValue=32  ResetInput=off  SamplesPerFrame=1  Ts=1  CntDtype=double  HitDtype=Logical
  Detect Decrease : simulink/Logic and Bit Operations/Detect Decrease  vinit=0.0  OutDataTypeStr=boolean
  Detect Increase : simulink/Logic and Bit Operations/Detect Increase  vinit=0.0  OutDataTypeStr=boolean
  Detect Rise Positive : simulink/Logic and Bit Operations/Detect Rise Positive  vinit=0  OutDataTypeStr=boolean
  MinMax Running Resettable : simulink/Math Operations/MinMax Running Resettable  Function=max  vinit=0.0
  Subsystem : Subsystem
  Amplitude : Outport
  Logical_output : Outport  Port=2
  wires:
  Fw/1 -> Detect Decrease/1, Detect Rise Positive/1, MinMax Running Resettable/1
  MinMax Running Resettable/1 -> Subsystem/1(In1)
  Detect Rise Positive/1 -> MinMax Running Resettable/2
  Detect Decrease/1 -> Subsystem/Trigger
  Detect Increase/1 -> Counter/1
  Subsystem/1(Out1) -> Amplitude/1, Detect Increase/1
  Compare To Constant1/1 -> Logical_output/1
  Counter/1 -> Compare To Constant1/1

== system modelo_completo_codesys_final/Mass calculation/Subsystem1/Peak_theta_detection1/Subsystem ==
  In1 : Inport
  Trigger : TriggerPort  VariantControl=Variant  PortDimensions=1
  Out1 : Outport
  wires:
  In1/1 -> Out1/1

== system modelo_completo_codesys_final/sending_setpoint_mechanisim/Trajectoria vxt/Subsystem3/Resettable Subsystem ==
  In1 : Inport
  len_vector : Inport  Port=2
  Reset : ResetPort  DisableCoverage=on  ResetTriggerType=either
  MATLAB Function : MATLAB Function  TreatAsAtomicUnit=on
  Memory : Memory
  Scope : Scope
  Out1 : Outport
  wires:
  len_vector/1 -> MATLAB Function/1(len_vec)
  MATLAB Function/2(vt) -> Out1/1
  MATLAB Function/1(cont) -> Scope/1, Memory/1
  Memory/1 -> MATLAB Function/3(cont_i)
  In1/1 -> MATLAB Function/2(qd)

== system modelo_completo_codesys_final/sending_setpoint_mechanisim/Trajectoria vyt/Subsystem3/Resettable Subsystem ==
  In1 : Inport
  len_vector : Inport  Port=2
  Reset : ResetPort  DisableCoverage=on  ResetTriggerType=either
  MATLAB Function : MATLAB Function  TreatAsAtomicUnit=on
  Memory : Memory
  Out1 : Outport
  wires:
  In1/1 -> MATLAB Function/2(qd)
  MATLAB Function/2(vt) -> Out1/1
  Memory/1 -> MATLAB Function/3(cont_i)
  MATLAB Function/1(cont) -> Memory/1
  len_vector/1 -> MATLAB Function/1(len_vec)

== system modelo_completo_codesys_final/sending_setpoint_mechanisim/Trajectoria vyt1/Subsystem3/Resettable Subsystem ==
  In1 : Inport
  len_vector : Inport  Port=2
  Reset : ResetPort  DisableCoverage=on  ResetTriggerType=either
  MATLAB Function : MATLAB Function  TreatAsAtomicUnit=on
  Memory : Memory
  Out1 : Outport
  wires:
  len_vector/1 -> MATLAB Function/1(len_vec)
  MATLAB Function/2(vt) -> Out1/1
  MATLAB Function/1(cont) -> Memory/1
  Memory/1 -> MATLAB Function/3(cont_i)
  In1/1 -> MATLAB Function/2(qd)

== system modelo_completo_codesys_final/sending_setpoint_mechanisim/Trajectoria vyt3/Subsystem3/Resettable Subsystem ==
  In1 : Inport
  len_vector : Inport  Port=2
  Reset : ResetPort  DisableCoverage=on  ResetTriggerType=either
  MATLAB Function : MATLAB Function  TreatAsAtomicUnit=on
  Memory : Memory
  Out1 : Outport
  wires:
  len_vector/1 -> MATLAB Function/1(len_vec)
  MATLAB Function/2(vt) -> Out1/1
  MATLAB Function/1(cont) -> Memory/1
  Memory/1 -> MATLAB Function/3(cont_i)
  In1/1 -> MATLAB Function/2(qd)

== system modelo_completo_codesys_final/Mass calculation/Subsystem/Subsystem/Peak_theta_detection1/Subsystem ==
  In1 : Inport
  Trigger : TriggerPort  VariantControl=Variant  PortDimensions=1
  Out1 : Outport
  wires:
  In1/1 -> Out1/1

== matlab function modelo_completo_codesys_final/Theta controller/Ganancias control theta ==
  data: Mt input; ml input; Kp output; Kd output; Wn input; lh input
function [Kp,Kd] = fcn(Mt,ml,Wn,lh)
    wpos = Wn*0.89;
    g=9.81;
    Kd = -lh + ( (Mt*g)/((wpos^2)*(ml+Mt)) ) ;
    Kp = 2*wpos*1*(lh + Kd);
end

== matlab function modelo_completo_codesys_final/sending_setpoint_mechanisim/Trajectoria vxt/Subsystem3/Resettable Subsystem/MATLAB Function ==
  data: len_vec input; qd input size=20000000,1; cont_i input; cont output; vt output
 function [cont, vt] = fcn(len_vec, qd,cont_i)
 if (cont_i<len_vec)
   cont=cont_i+1;
   vt = qd(cont,1);
 else
  vt = 0;
  cont=inf;
 end
 end

== matlab function modelo_completo_codesys_final/sending_setpoint_mechanisim/Trajectoria vyt/Subsystem3/Resettable Subsystem/MATLAB Function ==
  data: len_vec input; qd input size=20000000,1; cont_i input; cont output; vt output
 function [cont, vt] = fcn(len_vec, qd,cont_i)
 if (cont_i<len_vec)
   cont=cont_i+1;
   vt = qd(cont,1);
 else
  vt = 0;
  cont=inf;
 end
 end

== matlab function modelo_completo_codesys_final/sending_setpoint_mechanisim/Trajectoria vyt1/Subsystem3/Resettable Subsystem/MATLAB Function ==
  data: len_vec input; qd input size=20000000,1; cont_i input; cont output; vt output
 function [cont, vt] = fcn(len_vec, qd,cont_i)
 if (cont_i<len_vec)
   cont=cont_i+1;
   vt = qd(cont,1);
 else
  vt = 0;
  cont=inf;
 end
 end

== matlab function modelo_completo_codesys_final/sending_setpoint_mechanisim/Trajectoria vyt3/Subsystem3/Resettable Subsystem/MATLAB Function ==
  data: len_vec input; qd input size=20000000,1; cont_i input; cont output; vt output
 function [cont, vt] = fcn(len_vec, qd,cont_i)
 if (cont_i<len_vec)
   cont=cont_i+1;
   vt = qd(cont,1);
 else
  vt = 0;
  cont=inf;
 end
 end

== matlab function modelo_completo_codesys_final/MATLAB Function ==
  data: xl0 input; base_height output; boat_state input
function base_height    = get_base_height(xl0,boat_state)

boat_wide = 6;
boat_under_water = 10;
hy_cont = 2.5;


x_positions = [1.42,4.06,6.7,9.34,11.98,14.62];

if(xl0>=0)
posx_init_index = 1;
for i=1:boat_wide
    if(abs(xl0 - x_positions(i)) <= (2.44/2) + 0.1)
        posx_init_index = i;
    end
end

base_height=boat_state(posx_init_index)*hy_cont - boat_under_water;
else
base_height = hy_cont;  
posx_init_index=0;
end

end

== stateflow chart modelo_completo_codesys_final/Chart ==
  state Traj_generator
    state to_boat
      entry:  [vyt,vxt,xend,vx_end,vy_end,len,len2,nx_state] = gen_traj_boat(Boat_State,xl0,yl0,x_cointainer_setpoint,Load_state,Total_mass);
      vx_t=vxt; vy_t=vyt;vxend_t=vx_end;vyend_t=vy_end;len_out=len;len_out2 = len2;Boat_State=nx_state;
    state off
    state to_dock
      entry: [vyt,vxt,xend,vx_end,vy_end,len,len2,nx_state] = gen_traj_dock(Boat_State,xl0,yl0,1,Load_state,Total_mass);
      vx_t=vxt; vy_t=vyt;vxend_t=vx_end;vyend_t=vy_end; len_out=len; len_out2 = len2;Boat_State=nx_state;
    state to_dock1
      entry:  [vyt,vxt,xend,vx_end,vy_end,len,len2,nx_state] = gen_traj_cont_cont(Boat_State,xl0,yl0,x_cointainer_setpoint,Load_state,Total_mass);
      vx_t=vxt; vy_t=vyt;vxend_t=vx_end;vyend_t=vy_end;len_out=len;len_out2 = len2;Boat_State=nx_state;
    (default) -> off
    to_boat -> off : [~flag_gen_traj_boat]
    off -> to_boat [order 1] : [flag_gen_traj_boat]
    to_dock1 -> off : [~flag_gen_traj_cont]
    off -> to_dock1 [order 3] : [flag_gen_traj_cont]
    to_dock -> off : [~flag_gen_traj_dock]
    off -> to_dock [order 2] : [flag_gen_traj_dock]
  (default) -> Traj_generator
  data: estado_barco function_input; posx_init function_input; posy_init function_input; posx_end function_input; twistlocks function_input; vdyt function_output; vdxt function_output; x_end function_output; vxt_end function_output; vyt_end function_output; ml function_input; lenght function_output; lenght2 function_output; next_state function_output; estado_barco function_input; posx_init function_input; posy_init function_input; posx_end function_input; twistlocks function_input; vdyt function_output; vdxt function_output; x_end function_output; vxt_end function_output; vyt_end function_output; ml function_input; lenght function_output; lenght2 function_output; next_state function_output; estado_barco function_input; posx_init function_input; posy_init function_input; posx_end function_input; twistlocks function_input; vdyt function_output; vdxt function_output; x_end function_output; vxt_end function_output; vyt_end function_output; ml function_input; lenght function_output; lenght2 function_output; next_state function_output; xl0 input; yl0 input; xend output; vyend_t output size=20000000,1; vy_t output size=20000000,1; len_out2 output; len_out output; vx_t output size=20000000,1; vxend_t output size=20000000,1; Boat_State data_store_memory; vyt local size=20000000,1; len local; vy_end local size=20000000,1; vx_end local size=20000000,1; len2 local; nx_state local; vxt local size=20000000,1; Total_mass data_store_memory; Load_state data_store_memory; flag_gen_traj_boat input; flag_gen_traj_dock input; x_cointainer_setpoint data_store_memory; flag_gen_traj_cont input
  function [vdyt,vdxt,x_end,vxt_end,vyt_end,lenght,lenght2,next_state] = gen_traj_cont_cont(estado_barco,posx_init,posy_init,posx_end,twistlocks,ml):
    | function [vdyt,vdxt,x_end,vxt_end,vyt_end,lenght,lenght2,next_state] = gen_traj_cont_cont(estado_barco,posx_init,posy_init,posx_end,twistlocks,ml)
    | coder.extrinsic('cont_to_cont');
    | vdyt = [];
    | vdxt = [];
    | vxt_end =[];
    | vyt_end = [];
    | next_state=[0;0;0;0;0;0];
    | x_end=0;
    | lenght = 0;
    | lenght2 = 0;
    | coder.varsize('vdyt', [20000000 1]);
    | coder.varsize('vdxt', [20000000 1]);
    | coder.varsize('vyt_end', [20000000 1]);
    | coder.varsize('vxt_end', [20000000 1]);
    | [vdyt,vdxt,x_end,vxt_end,vyt_end,lenght,lenght2,next_state]=cont_to_cont(estado_barco,posx_init,posy_init,posx_end,twistlocks,ml);
    | end
  function [vdyt,vdxt,x_end,vxt_end,vyt_end,lenght,lenght2,next_state] = gen_traj_boat(estado_barco,posx_init,posy_init,posx_end,twistlocks,ml):
    | function [vdyt,vdxt,x_end,vxt_end,vyt_end,lenght,lenght2,next_state] = gen_traj_boat(estado_barco,posx_init,posy_init,posx_end,twistlocks,ml)
    | coder.extrinsic('gen_traj_to_boat');
    | vdyt = [];
    | vdxt = [];
    | vxt_end =[];
    | vyt_end = [];
    | next_state = [0; 0; 0; 0; 0; 0];
    | x_end=0;
    | lenght=0;
    | lenght2=0;
    | coder.varsize('vdyt', [20000000 1]);
    | coder.varsize('vdxt', [20000000 1]);
    | coder.varsize('vyt_end', [20000000 1]);
    | coder.varsize('vxt_end', [20000000 1]);
    | [vdyt,vdxt,x_end,vxt_end,vyt_end,lenght,lenght2,next_state]=gen_traj_to_boat(estado_barco,posx_init,posy_init,posx_end,twistlocks, ml);
    | end
  function [vdyt,vdxt,x_end,vxt_end,vyt_end,lenght,lenght2,next_state] = gen_traj_dock(estado_barco,posx_init,posy_init,posx_end,twistlocks,ml):
    | function [vdyt,vdxt,x_end,vxt_end,vyt_end,lenght,lenght2,next_state] = gen_traj_dock(estado_barco,posx_init,posy_init,posx_end,twistlocks,ml)
    | coder.extrinsic('gen_traj_to_dock');
    | vdyt = [];
    | vdxt = [];
    | vxt_end =[];
    | vyt_end = [];
    | x_end=0;
    | lenght=0;
    | lenght2 = 0;
    | next_state = [0;0;0;0;0;0];
    | coder.varsize('vdyt', [20000000 1]);
    | coder.varsize('vdxt', [20000000 1]);
    | coder.varsize('vyt_end', [20000000 1]);
    | coder.varsize('vxt_end', [20000000 1]);
    | [vdyt,vdxt,x_end,vxt_end,vyt_end,lenght,lenght2,next_state]=gen_traj_to_dock(estado_barco,posx_init,posy_init,posx_end,twistlocks,ml);
    | end
